simulink model "ball_balancing_omni3_multibody_lqi"  (R2026a)
settings: Solver=ode15s  StopTime=ballbotParams.simulation.stopTime  MaxStep=ballbotParams.simulation.maxStep  RelTol=ballbotParams.simulation.relativeTolerance
PreLoadFcn:
  | ballbotParams = ballbotParameters;
undefined symbols (not defined in the file or in its folder): ballbotEstimatorInitialState, ballbotEstimatorUpdate, ballbotImuFromJoint, ballbotLqiControllerUpdate, ballbotPoseFromJoint, ballbotServoVoltageController, ballbotWheelRateFromDisplacement, X, Y, Z
libraries: nesl_utility x38, sm_lib x26, fl_lib x12, ee_lib x3
(part 1 of 3)
settings Model: Creator=cafdr  LastModifiedBy=cafdr
settings SimscapeCC: SimscapeLogType=none

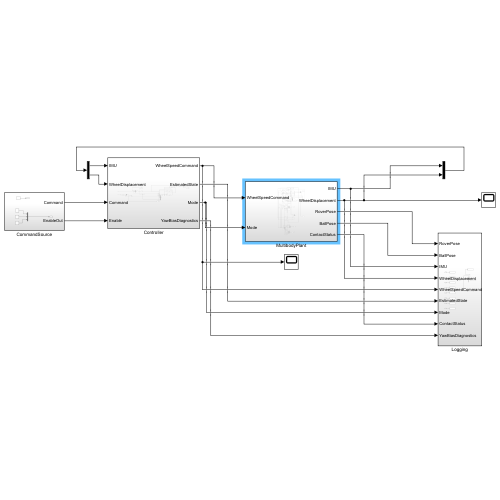
[thumbnail: Simulink's stored preview of the top-level diagram]
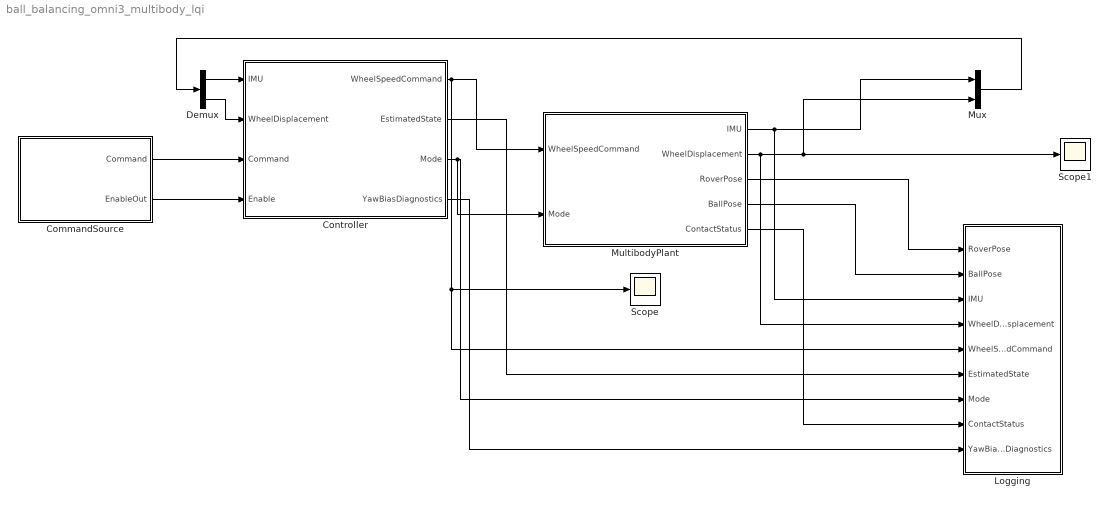
== system ball_balancing_omni3_multibody_lqi ==
  CommandSource : Subsystem
  Controller : Subsystem
  Demux : Demux  Outputs=2
  Logging : Subsystem
  MultibodyPlant : Subsystem
  Mux : Mux  Inputs=2
  Scope : Scope
      settings: ActiveDisplayYMinimum=-0.093711621357693731  ActiveDisplayYMaximum=0.065982668597649563
  Scope1 : Scope
      settings: ActiveDisplayYMinimum=-51.436545972709716  ActiveDisplayYMaximum=52.142033223021834
  wires:
  CommandSource/2(EnableOut) -> Controller/4(Enable)
  CommandSource/1(Command) -> Controller/3(Command)
  Mux/1 -> Demux/1
  Demux/1 -> Controller/1(IMU)
  Demux/2 -> Controller/2(WheelDisplacement)
  Controller/4(YawBiasDiagnostics) -> Logging/9(YawBiasDiagnostics)
  Controller/2(EstimatedState) -> Logging/6(EstimatedState)
  MultibodyPlant/5(ContactStatus) -> Logging/8(ContactStatus)
  Controller/3(Mode) -> Logging/7(Mode), MultibodyPlant/2(Mode)
  MultibodyPlant/4(BallPose) -> Logging/2(BallPose)
  MultibodyPlant/3(RoverPose) -> Logging/1(RoverPose)
  Controller/1(WheelSpeedCommand) -> Scope/1, Logging/5(WheelSpeedCommand), MultibodyPlant/1(WheelSpeedCommand)
  MultibodyPlant/1(IMU) -> Logging/3(IMU), Mux/1
  MultibodyPlant/2(WheelDisplacement) -> Mux/2, Scope1/1, Logging/4(WheelDisplacement)

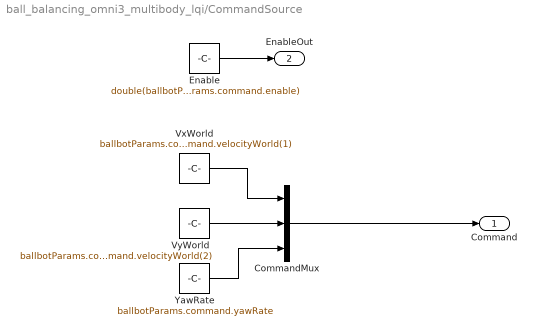
== system ball_balancing_omni3_multibody_lqi/CommandSource ==
  CommandMux : Mux  Inputs=3
  Enable : Constant  Value=double(ballbotParams.command.enable)  SampleTime=ballbotParams.controller.sampleTime
  VxWorld : Constant  Value=ballbotParams.command.velocityWorld(1)  SampleTime=ballbotParams.controller.sampleTime
  VyWorld : Constant  Value=ballbotParams.command.velocityWorld(2)  SampleTime=ballbotParams.controller.sampleTime
  YawRate : Constant  Value=ballbotParams.command.yawRate  SampleTime=ballbotParams.controller.sampleTime
  Command : Outport
  EnableOut : Outport  Port=2
  wires:
  Enable/1 -> EnableOut/1
  YawRate/1 -> CommandMux/3
  VxWorld/1 -> CommandMux/1
  VyWorld/1 -> CommandMux/2
  CommandMux/1 -> Command/1

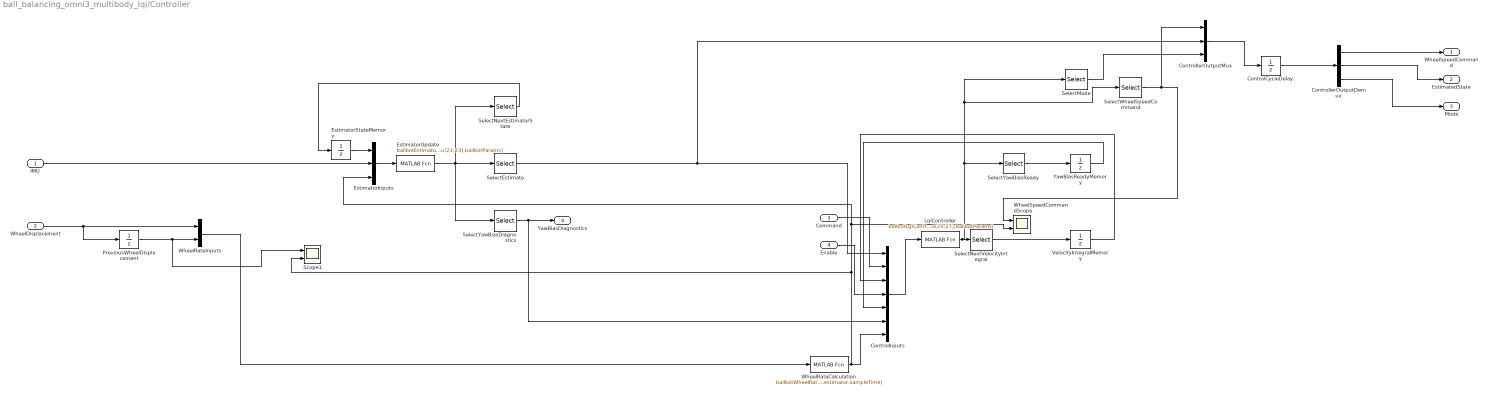
== system ball_balancing_omni3_multibody_lqi/Controller ==
  IMU : Inport  PortDimensions=6
  WheelDisplacement : Inport  Port=2  PortDimensions=3
  Command : Inport  Port=3
  Enable : Inport  Port=4
  ControlCycleDelay : UnitDelay  InitialCondition=zeros(18,1)  SampleTime=ballbotParams.controller.sampleTime
  ControlInputs : Mux  Inputs=7
  ControllerOutputDemux : Demux  Outputs=[3 14 1]
  ControllerOutputMux : Mux  Inputs=3
  EstimatorInputs : Mux  Inputs=3
  EstimatorStateMemory : UnitDelay  InitialCondition=ballbotEstimatorInitialState  SampleTime=ballbotParams.controller.sampleTime
  EstimatorUpdate : MATLABFcn  MATLABFcn=ballbotEstimatorUpdate(u(1:14),u(15:20),u(21:23),ballbotParams)  OutputDimensions=31  SampleTime=ballbotParams.controller.sampleTime
  LqiController : MATLABFcn  MATLABFcn=ballbotLqiControllerUpdate(u(1:14),u(15:17),u(18:19),u(20),u(21),u(22:24),u(25:27),ballbotParams)  OutputDimensions=7  SampleTime=ballbotParams.controller.sampleTime
  PreviousWheelDisplacement : UnitDelay  InitialCondition=zeros(3,1)  SampleTime=ballbotParams.controller.sampleTime
  Scope1 : Scope  NumInputPorts=2
      settings: ActiveDisplayYMinimum=-29.766814569729064  ActiveDisplayYMaximum=10.416225049193823  DataLoggingVariableName=ScopeData3
  SelectEstimate : Selector  InputPortWidth=31  IndexOptions=Index vector (dialog)  Indices=15:28  OutputSizes=1
  SelectMode : Selector  InputPortWidth=7  IndexOptions=Index vector (dialog)  Indices=6  OutputSizes=1
  SelectNextEstimatorState : Selector  InputPortWidth=31  IndexOptions=Index vector (dialog)  Indices=1:14  OutputSizes=1
  SelectNextVelocityIntegral : Selector  InputPortWidth=7  IndexOptions=Index vector (dialog)  Indices=4:5  OutputSizes=1
  SelectWheelSpeedCommand : Selector  InputPortWidth=7  IndexOptions=Index vector (dialog)  Indices=1:3  OutputSizes=1
  SelectYawBiasDiagnostics : Selector  InputPortWidth=31  IndexOptions=Index vector (dialog)  Indices=29:31  OutputSizes=1
  SelectYawBiasReady : Selector  InputPortWidth=7  IndexOptions=Index vector (dialog)  Indices=7  OutputSizes=1
  VelocityIntegralMemory : UnitDelay  InitialCondition=zeros(2,1)  SampleTime=ballbotParams.controller.sampleTime
  WheelRateCalculation : MATLABFcn  MATLABFcn=ballbotWheelRateFromDisplacement(u(1:3),u(4:6),ballbotParams.estimator.sampleTime)  OutputDimensions=3  SampleTime=ballbotParams.controller.sampleTime
  WheelRateInputs : Mux  Inputs=2
  WheelSpeedCommandScope : Scope  NumInputPorts=2
      settings: ActiveDisplayYMinimum=-1  ActiveDisplayYMaximum=1  DataLoggingVariableName=ScopeData2
  YawBiasReadyMemory : UnitDelay  SampleTime=ballbotParams.controller.sampleTime
  WheelSpeedCommand : Outport
  EstimatedState : Outport  Port=2
  Mode : Outport  Port=3
  YawBiasDiagnostics : Outport  Port=4
  wires:
  SelectNextEstimatorState/1 -> EstimatorStateMemory/1
  EstimatorInputs/1 -> EstimatorUpdate/1
  IMU/1 -> EstimatorInputs/2
  EstimatorStateMemory/1 -> EstimatorInputs/1
  PreviousWheelDisplacement/1 -> Scope1/1, WheelRateInputs/2
  WheelDisplacement/1 -> PreviousWheelDisplacement/1, WheelRateInputs/1
  ControlCycleDelay/1 -> ControllerOutputDemux/1
  ControllerOutputDemux/3 -> Mode/1
  ControllerOutputDemux/1 -> WheelSpeedCommand/1
  ControllerOutputDemux/2 -> EstimatedState/1
  EstimatorUpdate/1 -> SelectNextEstimatorState/1, SelectEstimate/1, SelectYawBiasDiagnostics/1
  SelectYawBiasReady/1 -> YawBiasReadyMemory/1
  ControlInputs/1 -> LqiController/1
  Enable/1 -> ControlInputs/4
  VelocityIntegralMemory/1 -> ControlInputs/3
  Command/1 -> ControlInputs/2
  SelectEstimate/1 -> ControlInputs/1, ControllerOutputMux/2
  SelectYawBiasDiagnostics/1 -> ControlInputs/6, YawBiasDiagnostics/1
  YawBiasReadyMemory/1 -> ControlInputs/5
  ControllerOutputMux/1 -> ControlCycleDelay/1
  SelectMode/1 -> ControllerOutputMux/3
  WheelRateInputs/1 -> WheelRateCalculation/1
  SelectWheelSpeedCommand/1 -> WheelSpeedCommandScope/1, ControllerOutputMux/1
  WheelRateCalculation/1 -> EstimatorInputs/3, WheelSpeedCommandScope/2, Scope1/2, ControlInputs/7
  LqiController/1 -> SelectMode/1, SelectWheelSpeedCommand/1, SelectYawBiasReady/1, SelectNextVelocityIntegral/1
  SelectNextVelocityIntegral/1 -> VelocityIntegralMemory/1

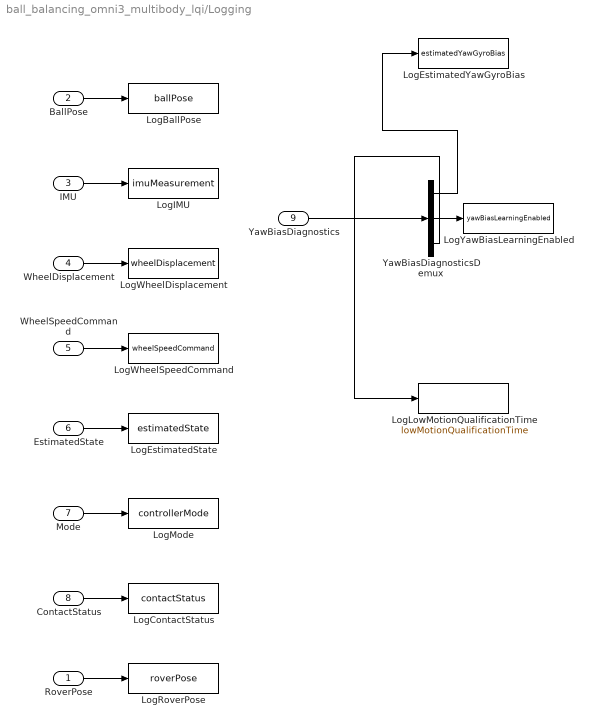
== system ball_balancing_omni3_multibody_lqi/Logging ==
  RoverPose : Inport
  BallPose : Inport  Port=2
  IMU : Inport  Port=3
  WheelDisplacement : Inport  Port=4
  WheelSpeedCommand : Inport  Port=5
  EstimatedState : Inport  Port=6
  Mode : Inport  Port=7
  ContactStatus : Inport  Port=8
  YawBiasDiagnostics : Inport  Port=9
  LogBallPose : ToWorkspace  VariableName=ballPose  SaveFormat=Timeseries  SampleTime=-1
  LogContactStatus : ToWorkspace  VariableName=contactStatus  SaveFormat=Timeseries  SampleTime=-1
  LogEstimatedState : ToWorkspace  VariableName=estimatedState  SaveFormat=Timeseries  SampleTime=-1
  LogEstimatedYawGyroBias : ToWorkspace  VariableName=estimatedYawGyroBias  SaveFormat=Timeseries  SampleTime=-1
  LogIMU : ToWorkspace  VariableName=imuMeasurement  SaveFormat=Timeseries  SampleTime=-1
  LogLowMotionQualificationTime : ToWorkspace  VariableName=lowMotionQualificationTime  SaveFormat=Timeseries  SampleTime=-1
  LogMode : ToWorkspace  VariableName=controllerMode  SaveFormat=Timeseries  SampleTime=-1
  LogRoverPose : ToWorkspace  VariableName=roverPose  SaveFormat=Timeseries  SampleTime=-1
  LogWheelDisplacement : ToWorkspace  VariableName=wheelDisplacement  SaveFormat=Timeseries  SampleTime=-1
  LogWheelSpeedCommand : ToWorkspace  VariableName=wheelSpeedCommand  SaveFormat=Timeseries  SampleTime=-1
  LogYawBiasLearningEnabled : ToWorkspace  VariableName=yawBiasLearningEnabled  SaveFormat=Timeseries  SampleTime=-1
  YawBiasDiagnosticsDemux : Demux  Outputs=3
  wires:
  ContactStatus/1 -> LogContactStatus/1
  Mode/1 -> LogMode/1
  EstimatedState/1 -> LogEstimatedState/1
  WheelSpeedCommand/1 -> LogWheelSpeedCommand/1
  WheelDisplacement/1 -> LogWheelDisplacement/1
  IMU/1 -> LogIMU/1
  BallPose/1 -> LogBallPose/1
  RoverPose/1 -> LogRoverPose/1
  YawBiasDiagnosticsDemux/3 -> LogLowMotionQualificationTime/1
  YawBiasDiagnosticsDemux/2 -> LogYawBiasLearningEnabled/1
  YawBiasDiagnosticsDemux/1 -> LogEstimatedYawGyroBias/1
  YawBiasDiagnostics/1 -> YawBiasDiagnosticsDemux/1
